simulink model "VehicleModel"  (R2016b)
settings: Solver=FixedStepAuto  StartTime=0.0  StopTime=t_EndSimulation  FixedStep=base_dT  MaxStep=0.01  RelTol=1e-3  EnableMultiTasking=on
values from neighbouring files (symbols this model uses):
  b_E2C_inloop = Simulink.Parameter    [VehicleModelInit.m]
  b_Engine_in_loop = Simulink.Parameter    [VehicleModelInit.m]
  b_initialize_distance_t_startsim = Simulink.Parameter    [VehicleModelInit.m]
  b_Ne_in_loop = Simulink.Parameter    [VehicleModelInit.m]
  b_TTB_in_loop = Simulink.Parameter    [VehicleModelInit.m]
  b_use_acc = Simulink.Parameter    [VehicleModelInit.m]
  b_use_acc_hardset = Simulink.Parameter    [VehicleModelInit.m]
  base_dT = Simulink.Parameter    [VehicleModelInit.m]
  c_acc_d_hdw = Simulink.Parameter    [VehicleModelInit.m]
  c_acc_hdw = Simulink.Parameter    [VehicleModelInit.m]
  c_EngFricCoef = PARS.c_EngFricCoef    [VehicleModelInit.m]
  c_EngFricCoefd = PARS.c_EngFricCoefd    [VehicleModelInit.m]
  d_Ne_max = Simulink.Parameter    [VehicleModelInit.m]
  d_Ne_min = Simulink.Parameter    [VehicleModelInit.m]
  Driver_TuneG1 = PARS.Driver_TuneG1    [VehicleModelInit.m]
  Driver_TuneG2 = PARS.Driver_TuneG2    [VehicleModelInit.m]
  Driver_TuneG3 = PARS.Driver_TuneG3    [VehicleModelInit.m]
  Driver_TuneG_aw = PARS.Driver_TuneG_aw    [VehicleModelInit.m]
  E2C_c2_dTB = Simulink.Parameter    [VehicleModelInit.m]
  E2C_c_dTB = Simulink.Parameter    [VehicleModelInit.m]
  E2C_CycleTimespan = Simulink.Parameter    [VehicleModelInit.m]
  E2C_initializeRelDist = Simulink.Parameter    [VehicleModelInit.m]
  E2C_SpeedShape = Simulink.Parameter    [VehicleModelInit.m]
  E2C_Trap_CycleAcceEndAlpha = Simulink.Parameter    [VehicleModelInit.m]
  E2C_Trap_CycleAcceStartAlpha = Simulink.Parameter    [VehicleModelInit.m]
  E2C_Trap_CycleDeceEndAlpha = Simulink.Parameter    [VehicleModelInit.m]
  E2C_Trap_CycleDeceStartAlpha = Simulink.Parameter    [VehicleModelInit.m]
  E2C_V_High_kmh = Simulink.Parameter    [VehicleModelInit.m]
  E2C_V_Low_kmh = Simulink.Parameter    [VehicleModelInit.m]
  E2C_V_max = Simulink.Parameter    [VehicleModelInit.m]
  E2C_V_min = Simulink.Parameter    [VehicleModelInit.m]
  FTP_speed_1sec = [FTP_speed_once.speed;Idle_speed_once;FTP_speed_once.speed;Idle_speed_once;FTP_speed_once.speed]    [VehicleModelInit.m]
  mass = 3123*1.3    (= 4059.9)    [VehicleModelInit.m]
  T_ACC_TuneG1_data = Simulink.Parameter    [VehicleModelInit.m]
  T_ACC_TuneG1_pt = Simulink.Parameter    [VehicleModelInit.m]
  T_ACC_TuneG2_data = Simulink.Parameter    [VehicleModelInit.m]
  T_ACC_TuneG2_pt = Simulink.Parameter    [VehicleModelInit.m]
  t_StartSimulation = Simulink.Parameter    [VehicleModelInit.m]
  T_TB_ego_ini = Simulink.Parameter    [VehicleModelInit.m]
  T_TB_OffSet = Simulink.Parameter    [VehicleModelInit.m]
  tau_EngTorque = Simulink.Parameter    [VehicleModelInit.m]
  tau_Ne = Simulink.Parameter    [VehicleModelInit.m]
  tau_pedal_dem = Simulink.Parameter    [VehicleModelInit.m]
  VESP_MD = x0.VESP    [VehicleModelInit.m]
undefined symbols (not defined in the file or in its folder): Continuous, DiscIntNeverNeededParam, initializeRelDist, p_ego_ini, p_lead_ini, PedalMapMD, r_w, Simulation_dT, spsSampleAndHoldModel, v_lead_ini, x0
libraries: simulink x9, spsEdgeDetectorModel x6, dspsigops x1
(part 4 of 7)

== matlab function VehicleModel/Subsystem/Follower vehicle Subsystem/Follow Vehicle/Vehicle Resistance Model ==
  data: Frol output; Fd output; VESP_mph input; Grade_deg input; F_res output; B_pedal input; Mass input; Cr input; Cw input; Aa input; Fb output
function [Frol,Fd,F_res,Fb] =VehModel(VESP_mph,Grade_deg,B_pedal,Mass,Cr,Cw,Aa)
%Grade is in Deg VESP is in MPH
mass = Mass; 
c_w  = Cw;
A_a  = Aa;
% i_f = 3.4;
% r_w = 0.57; % For M915A3 tracotr
%Drive conditions
rho=1.0; % Air density
%VESP=VESP_init./2.23694; %initial vehicle speed
% i_t=gears_ratios(G_level); % Gear ratio
Fg=mass*9.81*sin(Grade_deg*pi/180); % Fgrade force with grade in degree
%Fe=Tq/r_w*(i_t*i_f); % Engine force
%Ftrac=(Fe-Fg-Fr-Fd);
Fd=0.5*c_w*A_a*rho*(VESP_mph/2.23694)^2;  %Drag force
Fb=B_pedal*100e3; %Brake force
Frol = mass*9.81*Cr;
F_res=(Fd+Frol+Fg+Fb);
